simulink model "ES320A_MotDrvDiagc"  (R2013b)
settings: Solver=FixedStepDiscrete  StartTime=0.0  StopTime=1  FixedStep=.002  RelTol=1e-3
undefined symbols (not defined in the file): ARCHGLBPRM_2MILLISEC_SEC_F32, MotDrvDiagcErrFilFrq, MotDrvDiagcErrOffs, MotDrvDiagcErrThd, NtcNr1, NtcSts1, PHAONTISUMMAX_NANOSEC_U32, SysSt1
libraries: simulink x23, Fil x12, NxtrAbslt x6, NxtrLim x6
(part 2 of 3)

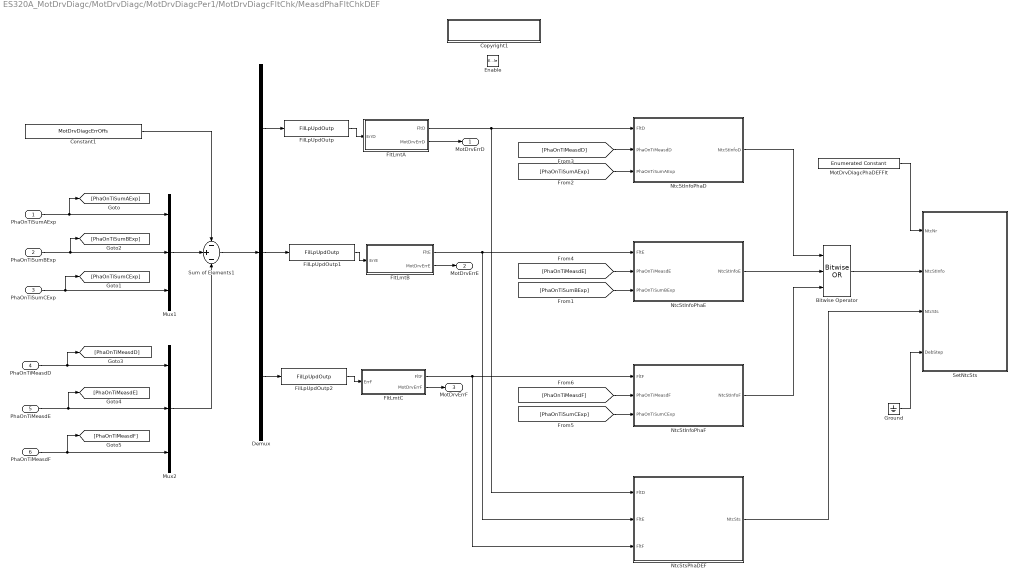
== system ES320A_MotDrvDiagc/MotDrvDiagc/MotDrvDiagcPer1/MotDrvDiagcFltChk/MeasdPhaFltChkDEF ==
  PhaOnTiSumAExp : Inport
  PhaOnTiSumBExp : Inport  Port=2
  PhaOnTiSumCExp : Inport  Port=3
  PhaOnTiMeasdD : Inport  Port=4
  PhaOnTiMeasdE : Inport  Port=5
  PhaOnTiMeasdF : Inport  Port=6
  Enable : EnablePort  StatesWhenEnabling=reset
  Bitwise Operator : simulink/Logic and Bit Operations/Bitwise Operator  logicop=OR  UseBitMask=off  NumInputPorts=3  BitMask=bin2dec('11011001')  BitMaskRealWorld=Stored Integer
  Constant1 : Constant  Value=MotDrvDiagcErrOffs
  Copyright1 : Subsystem  Description=|  RequirementInfo={} %GIDa_58fa1417_7a97_4da9_9225_f2d3186cfd6f  mask(Copyright Information){none=on}
      | Copyright info block.                                               
      |                                                                     
      | Place copyright information at the top of every subsystem in design.
      mask prompts: none "No parameters"
      mask help: Place copyright information at the top of every subsystem in design.
      mask Display:
      | NxtrConf = 'Nexteer Confidential';
      | 
      | sys = bdroot; %handle for the current model ("system")
      | first = get_param(sys,'Created');
      | if(isempty(first))
      |     first = datestr(now,'yyyy');
      | else
      |     first = first(end-3:end);  %year is last four digits
      | end
      | 
      | last = get_param(sys,'LastModifiedDate');
      | if isempty(last)
      |     last = datestr(now,'yyyy');
      | else
      |     last = last(end-3:end);
      | end
      | 
      | if strcmp(first,last)
      |     fprintf('%s\nCopyright  %s Nexteer',NxtrConf,first);
      | else
      |     fprintf('%s\n%s%s-%s Nexteer',NxtrConf,char(169),first,last);
      | end
  Demux : Demux  Outputs=3
  FilLpUpdOutp : Fil/FilLpUpdOutp  StVar=MotDrvDiagcPhaDFilLp
      settings: AttributesFormatString=StVar: %<StVar>
  FilLpUpdOutp1 : Fil/FilLpUpdOutp  StVar=MotDrvDiagcPhaEFilLp
      settings: AttributesFormatString=StVar: %<StVar>
  FilLpUpdOutp2 : Fil/FilLpUpdOutp  StVar=MotDrvDiagcPhaFFilLp
      settings: AttributesFormatString=StVar: %<StVar>
  FltLmtA : Subsystem  RequirementInfo={'linktype_rmi_doors' '0000cf4c (/ESG Group/FDD Module Requirements/EA4 Specific/ES320A_MotDrvDiagc)' '#ES320A_212' 'true' 'REQ: ES320A_212' '' } %GIDa_51d7d654_d101_4f83_80bf_ae722de7e7a9
  FltLmtB : Subsystem  RequirementInfo={'linktype_rmi_doors' '0000cf4c (/ESG Group/FDD Module Requirements/EA4 Specific/ES320A_MotDrvDiagc)' '#ES320A_211' 'true' 'REQ: ES320A_211' '' } %GIDa_eddb3f9b_306c_4d4f_962f_9a75bcde932a
  FltLmtC : Subsystem  RequirementInfo={'linktype_rmi_doors' '0000cf4c (/ESG Group/FDD Module Requirements/EA4 Specific/ES320A_MotDrvDiagc)' '#ES320A_210' 'true' 'REQ: ES320A_210' '' } %GIDa_51c857d3_af1b_4868_8ae8_03f92acada51
  Ground : Ground
  MotDrvDiagcPhaDEFFlt : simulink/Sources/Enumerated Constant  OutDataTypeStr=Enum: NtcNr1  Value=NtcNr1.NTCNR_0X064  SampleTime=inf
  Mux1 : Mux  Inputs=3
  Mux2 : Mux  Inputs=3
  NtcStInfoPhaD : Subsystem
  NtcStInfoPhaE : Subsystem
  NtcStInfoPhaF : Subsystem
  NtcStsPhaDEF : Subsystem  RequirementInfo={'linktype_rmi_doors' '0000cf4c (/ESG Group/FDD Module Requirements/EA4 Specific/ES320A_MotDrvDiagc)' '#ES320A_202' 'true' 'REQ: ES320A_202' '' } %GIDa_66002cee_da6e_4218_8b0a_b4f0ffa61e1a
  SetNtcSts : Subsystem  RequirementInfo={'linktype_rmi_doors' '0000cf4c (/ESG Group/FDD Module Requirements/EA4 Specific/ES320A_MotDrvDiagc)' '#ES320A_159' 'true' 'REQ: ES320A_159' '' } %GIDa_c4017480_1c1a_46e6_ad44_3193a372f033
  Sum of Elements1 : Sum  Inputs=-+-  OutDataTypeStr=single
  MotDrvErrD : Outport
  MotDrvErrE : Outport  Port=2
  MotDrvErrF : Outport  Port=3
  wires:
  FltLmtA/1(FltD) -> NtcStsPhaDEF/1(FltD), NtcStInfoPhaD/1(FltD)
  FltLmtC/1(FltF) -> NtcStsPhaDEF/3(FltF), NtcStInfoPhaF/1(FltF)
  [PhaOnTiMeasdD] -> NtcStInfoPhaD/2(PhaOnTiMeasdD)
  [PhaOnTiSumAExp] -> NtcStInfoPhaD/3(PhaOnTiSumAExp)
  [PhaOnTiMeasdE] -> NtcStInfoPhaE/2(PhaOnTiMeasdE)
  [PhaOnTiSumBExp] -> NtcStInfoPhaE/3(PhaOnTiSumBExp)
  [PhaOnTiMeasdF] -> NtcStInfoPhaF/2(PhaOnTiMeasdF)
  [PhaOnTiSumCExp] -> NtcStInfoPhaF/3(PhaOnTiSumCExp)
  NtcStInfoPhaD/1(NtcStInfoD) -> Bitwise Operator/1
  NtcStInfoPhaE/1(NtcStInfoE) -> Bitwise Operator/2
  NtcStInfoPhaF/1(NtcStInfoF) -> Bitwise Operator/3
  FilLpUpdOutp/1 -> FltLmtA/1(ErrD)
  FilLpUpdOutp2/1 -> FltLmtC/1(ErrF)
  Bitwise Operator/1 -> SetNtcSts/2(NtcStInfo)
  NtcStsPhaDEF/1(NtcSts) -> SetNtcSts/3(NtcSts)
  PhaOnTiMeasdF/1 -> [PhaOnTiMeasdF], Mux2/3
  PhaOnTiMeasdE/1 -> [PhaOnTiMeasdE], Mux2/2
  PhaOnTiMeasdD/1 -> [PhaOnTiMeasdD], Mux2/1
  Constant1/1 -> Sum of Elements1/1
  Mux2/1 -> Sum of Elements1/3
  Sum of Elements1/1 -> Demux/1
  Mux1/1 -> Sum of Elements1/2
  PhaOnTiSumAExp/1 -> [PhaOnTiSumAExp], Mux1/1
  PhaOnTiSumCExp/1 -> [PhaOnTiSumCExp], Mux1/3
  PhaOnTiSumBExp/1 -> [PhaOnTiSumBExp], Mux1/2
  Demux/1 -> FilLpUpdOutp/1
  Demux/2 -> FilLpUpdOutp1/1
  Demux/3 -> FilLpUpdOutp2/1
  Ground/1 -> SetNtcSts/4(DebStep)
  MotDrvDiagcPhaDEFFlt/1 -> SetNtcSts/1(NtcNr)
  FltLmtB/1(FltE) -> NtcStsPhaDEF/2(FltE), NtcStInfoPhaE/1(FltE)
  FilLpUpdOutp1/1 -> FltLmtB/1(ErrE)
  FltLmtA/2(MotDrvErrD) -> MotDrvErrD/1
  FltLmtB/2(MotDrvErrE) -> MotDrvErrE/1
  FltLmtC/2(MotDrvErrF) -> MotDrvErrF/1

== system ES320A_MotDrvDiagc/MotDrvDiagc/MotDrvDiagcPer1/DeltaCompu/else/CopyRight1 ==

== system ES320A_MotDrvDiagc/MotDrvDiagc/MotDrvDiagcPer1/DeltaCompu/else1/CopyRight1 ==

== system ES320A_MotDrvDiagc/MotDrvDiagc/MotDrvDiagcPer1/DeltaCompu/else2/CopyRight1 ==

== system ES320A_MotDrvDiagc/MotDrvDiagc/MotDrvDiagcPer1/DeltaCompu/if/CopyRight1 ==

== system ES320A_MotDrvDiagc/MotDrvDiagc/MotDrvDiagcPer1/DeltaCompu/if1/CopyRight1 ==

== system ES320A_MotDrvDiagc/MotDrvDiagc/MotDrvDiagcPer1/DeltaCompu/if2/CopyRight1 ==

== system ES320A_MotDrvDiagc/MotDrvDiagc/MotDrvDiagcPer1/MotDrvDiagcFltChk/MeasdPhaFltChkABC/Copyright1 ==

== system ES320A_MotDrvDiagc/MotDrvDiagc/MotDrvDiagcPer1/MotDrvDiagcFltChk/MeasdPhaFltChkABC/FltLmtA ==
  ErrA : Inport
  Abslt_f32_f32 : NxtrAbslt/Abslt_f32_f32  SFunctionSpec=single y1 = Abslt_f32_f32(single u1)
      settings: AttributesFormatString=%<Name>
  Constant2 : Constant  Value=MotDrvDiagcErrThd
  Copyright1 : Subsystem  Description=|  RequirementInfo={} %GIDa_ded85060_8e2b_4f15_bbc9_ae7ad683cc8a  mask(Copyright Information){none=on}
      | Copyright info block.                                               
      |                                                                     
      | Place copyright information at the top of every subsystem in design.
      mask prompts: none "No parameters"
      mask help: Place copyright information at the top of every subsystem in design.
      mask Display:
      | NxtrConf = 'Nexteer Confidential';
      | 
      | sys = bdroot; %handle for the current model ("system")
      | first = get_param(sys,'Created');
      | if(isempty(first))
      |     first = datestr(now,'yyyy');
      | else
      |     first = first(end-3:end);  %year is last four digits
      | end
      | 
      | last = get_param(sys,'LastModifiedDate');
      | if isempty(last)
      |     last = datestr(now,'yyyy');
      | else
      |     last = last(end-3:end);
      | end
      | 
      | if strcmp(first,last)
      |     fprintf('%s\nCopyright  %s Nexteer',NxtrConf,first);
      | else
      |     fprintf('%s\n%s%s-%s Nexteer',NxtrConf,char(169),first,last);
      | end
  LimStat_f1 : NxtrLim/LimStat_f32  LoLim=MotDrvErrA.EngMin  HiLim=MotDrvErrA.EngMax
      settings: AttributesFormatString=|
      | Low Limit: %<LoLim>
      | High Limit:%<HiLim>
  Relational Operator : RelationalOperator  Operator=>  OutDataTypeStr=boolean
  FltA : Outport
  MotDrvErrA : Outport  Port=2
  wires:
  ErrA/1 -> Abslt_f32_f32/1
  Constant2/1 -> Relational Operator/2
  Relational Operator/1 -> FltA/1
  Abslt_f32_f32/1 -> LimStat_f1/1, Relational Operator/1
  LimStat_f1/1 -> MotDrvErrA/1

== system ES320A_MotDrvDiagc/MotDrvDiagc/MotDrvDiagcPer1/MotDrvDiagcFltChk/MeasdPhaFltChkABC/FltLmtB ==
  ErrB : Inport
  Abslt_f32_f32 : NxtrAbslt/Abslt_f32_f32  SFunctionSpec=single y1 = Abslt_f32_f32(single u1)
      settings: AttributesFormatString=%<Name>
  Constant2 : Constant  Value=MotDrvDiagcErrThd
  Copyright1 : Subsystem  Description=|  RequirementInfo={} %GIDa_76afdc08_624c_4107_8b02_e46a83163c5b  mask(Copyright Information){none=on}
      | Copyright info block.                                               
      |                                                                     
      | Place copyright information at the top of every subsystem in design.
      mask prompts: none "No parameters"
      mask help: Place copyright information at the top of every subsystem in design.
      mask Display:
      | NxtrConf = 'Nexteer Confidential';
      | 
      | sys = bdroot; %handle for the current model ("system")
      | first = get_param(sys,'Created');
      | if(isempty(first))
      |     first = datestr(now,'yyyy');
      | else
      |     first = first(end-3:end);  %year is last four digits
      | end
      | 
      | last = get_param(sys,'LastModifiedDate');
      | if isempty(last)
      |     last = datestr(now,'yyyy');
      | else
      |     last = last(end-3:end);
      | end
      | 
      | if strcmp(first,last)
      |     fprintf('%s\nCopyright  %s Nexteer',NxtrConf,first);
      | else
      |     fprintf('%s\n%s%s-%s Nexteer',NxtrConf,char(169),first,last);
      | end
  LimStat_f2 : NxtrLim/LimStat_f32  LoLim=MotDrvErrB.EngMin  HiLim=MotDrvErrB.EngMax
      settings: AttributesFormatString=|
      | Low Limit: %<LoLim>
      | High Limit:%<HiLim>
  Relational Operator : RelationalOperator  Operator=>  OutDataTypeStr=boolean
  FltB : Outport
  MotDrvErrB : Outport  Port=2
  wires:
  Relational Operator/1 -> FltB/1
  Constant2/1 -> Relational Operator/2
  Abslt_f32_f32/1 -> LimStat_f2/1, Relational Operator/1
  ErrB/1 -> Abslt_f32_f32/1
  LimStat_f2/1 -> MotDrvErrB/1

== system ES320A_MotDrvDiagc/MotDrvDiagc/MotDrvDiagcPer1/MotDrvDiagcFltChk/MeasdPhaFltChkABC/FltLmtC ==
  ErrC : Inport
  Abslt_f32_f32 : NxtrAbslt/Abslt_f32_f32  SFunctionSpec=single y1 = Abslt_f32_f32(single u1)
      settings: AttributesFormatString=%<Name>
  Constant2 : Constant  Value=MotDrvDiagcErrThd
  Copyright1 : Subsystem  Description=|  RequirementInfo={} %GIDa_37053073_c47e_4fb3_8cd7_4f83c0fb15a4  mask(Copyright Information){none=on}
      | Copyright info block.                                               
      |                                                                     
      | Place copyright information at the top of every subsystem in design.
      mask prompts: none "No parameters"
      mask help: Place copyright information at the top of every subsystem in design.
      mask Display:
      | NxtrConf = 'Nexteer Confidential';
      | 
      | sys = bdroot; %handle for the current model ("system")
      | first = get_param(sys,'Created');
      | if(isempty(first))
      |     first = datestr(now,'yyyy');
      | else
      |     first = first(end-3:end);  %year is last four digits
      | end
      | 
      | last = get_param(sys,'LastModifiedDate');
      | if isempty(last)
      |     last = datestr(now,'yyyy');
      | else
      |     last = last(end-3:end);
      | end
      | 
      | if strcmp(first,last)
      |     fprintf('%s\nCopyright  %s Nexteer',NxtrConf,first);
      | else
      |     fprintf('%s\n%s%s-%s Nexteer',NxtrConf,char(169),first,last);
      | end
  LimStat_f3 : NxtrLim/LimStat_f32  LoLim=MotDrvErrC.EngMin  HiLim=MotDrvErrC.EngMax
      settings: AttributesFormatString=|
      | Low Limit: %<LoLim>
      | High Limit:%<HiLim>
  Relational Operator : RelationalOperator  Operator=>  OutDataTypeStr=boolean
  FltC : Outport
  MotDrvErrC : Outport  Port=2
  wires:
  ErrC/1 -> Abslt_f32_f32/1
  Constant2/1 -> Relational Operator/2
  Relational Operator/1 -> FltC/1
  Abslt_f32_f32/1 -> LimStat_f3/1, Relational Operator/1
  LimStat_f3/1 -> MotDrvErrC/1

== system ES320A_MotDrvDiagc/MotDrvDiagc/MotDrvDiagcPer1/MotDrvDiagcFltChk/MeasdPhaFltChkABC/NtcStInfoPhaA ==
  FltA : Inport
  PhaOnTiMeasdA : Inport  Port=2
  PhaOnTiSumAExp : Inport  Port=3
  Copyright1 : Subsystem  Description=|  RequirementInfo={} %GIDa_f6b7d8fe_5be3_402f_916a_b6caca477132  mask(Copyright Information){none=on}
      | Copyright info block.                                               
      |                                                                     
      | Place copyright information at the top of every subsystem in design.
      mask prompts: none "No parameters"
      mask help: Place copyright information at the top of every subsystem in design.
      mask Display:
      | NxtrConf = 'Nexteer Confidential';
      | 
      | sys = bdroot; %handle for the current model ("system")
      | first = get_param(sys,'Created');
      | if(isempty(first))
      |     first = datestr(now,'yyyy');
      | else
      |     first = first(end-3:end);  %year is last four digits
      | end
      | 
      | last = get_param(sys,'LastModifiedDate');
      | if isempty(last)
      |     last = datestr(now,'yyyy');
      | else
      |     last = last(end-3:end);
      | end
      | 
      | if strcmp(first,last)
      |     fprintf('%s\nCopyright  %s Nexteer',NxtrConf,first);
      | else
      |     fprintf('%s\n%s%s-%s Nexteer',NxtrConf,char(169),first,last);
      | end
  DetermineBitsetA : Subsystem  TreatAsAtomicUnit=on
  DetermineBitsetA1 : Subsystem  RequirementInfo={'linktype_rmi_doors' '0000cf4c (/ESG Group/FDD Module Requirements/EA4 Specific/ES320A_MotDrvDiagc)' '#ES320A_164' 'true' 'REQ: ES320A_164' '' } %GIDa_a157fcae_4dcd_4f05_b388_763736355bda  TreatAsAtomicUnit=on
  If : If  IfExpression=u1 == 1
  Merge : Merge
  NtcStInfoA : Outport
  wires:
  PhaOnTiMeasdA/1 -> DetermineBitsetA/1(PhaOnTiMeasdA)
  DetermineBitsetA1/1(BitSetA) -> Merge/2
  FltA/1 -> If/1
  DetermineBitsetA/1(BitSetA) -> Merge/1
  PhaOnTiSumAExp/1 -> DetermineBitsetA/2(PhaOnTiSumAExp)
  Merge/1 -> NtcStInfoA/1
  If/1 -> DetermineBitsetA/Action
  If/2 -> DetermineBitsetA1/Action

== system ES320A_MotDrvDiagc/MotDrvDiagc/MotDrvDiagcPer1/MotDrvDiagcFltChk/MeasdPhaFltChkABC/NtcStInfoPhaB ==
  FltB : Inport
  PhaOnTiMeasdB : Inport  Port=2
  PhaOnTiSumBExp : Inport  Port=3
  Copyright1 : Subsystem  Description=|  RequirementInfo={} %GIDa_8a865a79_d063_4821_8f7f_5a173239adfd  mask(Copyright Information){none=on}
      | Copyright info block.                                               
      |                                                                     
      | Place copyright information at the top of every subsystem in design.
      mask prompts: none "No parameters"
      mask help: Place copyright information at the top of every subsystem in design.
      mask Display:
      | NxtrConf = 'Nexteer Confidential';
      | 
      | sys = bdroot; %handle for the current model ("system")
      | first = get_param(sys,'Created');
      | if(isempty(first))
      |     first = datestr(now,'yyyy');
      | else
      |     first = first(end-3:end);  %year is last four digits
      | end
      | 
      | last = get_param(sys,'LastModifiedDate');
      | if isempty(last)
      |     last = datestr(now,'yyyy');
      | else
      |     last = last(end-3:end);
      | end
      | 
      | if strcmp(first,last)
      |     fprintf('%s\nCopyright  %s Nexteer',NxtrConf,first);
      | else
      |     fprintf('%s\n%s%s-%s Nexteer',NxtrConf,char(169),first,last);
      | end
  DetermineBitsetB : Subsystem  TreatAsAtomicUnit=on
  DetermineBitsetB1 : Subsystem  RequirementInfo={'linktype_rmi_doors' '0000cf4c (/ESG Group/FDD Module Requirements/EA4 Specific/ES320A_MotDrvDiagc)' '#ES320A_164' 'true' 'REQ: ES320A_164' '' } %GIDa_ef53c142_7f27_4df6_aa45_b15ec14132a0  TreatAsAtomicUnit=on
  If : If  IfExpression=u1 == 1
  Merge : Merge
  NtcStInfoB : Outport
  wires:
  DetermineBitsetB1/1(BitSetB) -> Merge/2
  FltB/1 -> If/1
  PhaOnTiSumBExp/1 -> DetermineBitsetB/2(PhaOnTiSumBExp)
  PhaOnTiMeasdB/1 -> DetermineBitsetB/1(PhaOnTiMeasdB)
  Merge/1 -> NtcStInfoB/1
  DetermineBitsetB/1(BitSetB) -> Merge/1
  If/1 -> DetermineBitsetB/Action
  If/2 -> DetermineBitsetB1/Action

== system ES320A_MotDrvDiagc/MotDrvDiagc/MotDrvDiagcPer1/MotDrvDiagcFltChk/MeasdPhaFltChkABC/NtcStInfoPhaC ==
  FltC : Inport
  PhaOnTiMeasdC : Inport  Port=2
  PhaOnTiSumCExp : Inport  Port=3
  Copyright1 : Subsystem  Description=|  RequirementInfo={} %GIDa_1949ea6a_a67d_400f_aabf_09f17ca06aa3  mask(Copyright Information){none=on}
      | Copyright info block.                                               
      |                                                                     
      | Place copyright information at the top of every subsystem in design.
      mask prompts: none "No parameters"
      mask help: Place copyright information at the top of every subsystem in design.
      mask Display:
      | NxtrConf = 'Nexteer Confidential';
      | 
      | sys = bdroot; %handle for the current model ("system")
      | first = get_param(sys,'Created');
      | if(isempty(first))
      |     first = datestr(now,'yyyy');
      | else
      |     first = first(end-3:end);  %year is last four digits
      | end
      | 
      | last = get_param(sys,'LastModifiedDate');
      | if isempty(last)
      |     last = datestr(now,'yyyy');
      | else
      |     last = last(end-3:end);
      | end
      | 
      | if strcmp(first,last)
      |     fprintf('%s\nCopyright  %s Nexteer',NxtrConf,first);
      | else
      |     fprintf('%s\n%s%s-%s Nexteer',NxtrConf,char(169),first,last);
      | end
  DetermineBitsetC : Subsystem  TreatAsAtomicUnit=on
  DetermineBitsetC1 : Subsystem  RequirementInfo={'linktype_rmi_doors' '0000cf4c (/ESG Group/FDD Module Requirements/EA4 Specific/ES320A_MotDrvDiagc)' '#ES320A_164' 'true' 'REQ: ES320A_164' '' } %GIDa_512545ae_b061_4cfd_bb08_eb9229f95692  TreatAsAtomicUnit=on
  If : If  IfExpression=u1 == 1
  Merge : Merge
  NtcStInfoC : Outport
  wires:
  FltC/1 -> If/1
  PhaOnTiSumCExp/1 -> DetermineBitsetC/2(PhaOnTiSumCExp)
  PhaOnTiMeasdC/1 -> DetermineBitsetC/1(PhaOnTiMeasdC)
  DetermineBitsetC/1(BitSetC) -> Merge/1
  DetermineBitsetC1/1(BitSetC) -> Merge/2
  Merge/1 -> NtcStInfoC/1
  If/1 -> DetermineBitsetC/Action
  If/2 -> DetermineBitsetC1/Action

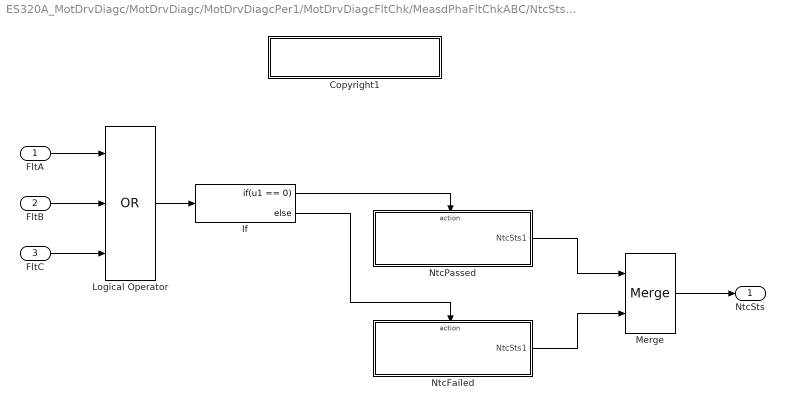
== system ES320A_MotDrvDiagc/MotDrvDiagc/MotDrvDiagcPer1/MotDrvDiagcFltChk/MeasdPhaFltChkABC/NtcStsPhaABC ==
  FltA : Inport
  FltB : Inport  Port=2
  FltC : Inport  Port=3
  Copyright1 : Subsystem  Description=|  RequirementInfo={} %GIDa_bbf24996_5a5d_487b_b234_27f9deb21f2d  mask(Copyright Information){none=on}
      | Copyright info block.                                               
      |                                                                     
      | Place copyright information at the top of every subsystem in design.
      mask prompts: none "No parameters"
      mask help: Place copyright information at the top of every subsystem in design.
      mask Display:
      | NxtrConf = 'Nexteer Confidential';
      | 
      | sys = bdroot; %handle for the current model ("system")
      | first = get_param(sys,'Created');
      | if(isempty(first))
      |     first = datestr(now,'yyyy');
      | else
      |     first = first(end-3:end);  %year is last four digits
      | end
      | 
      | last = get_param(sys,'LastModifiedDate');
      | if isempty(last)
      |     last = datestr(now,'yyyy');
      | else
      |     last = last(end-3:end);
      | end
      | 
      | if strcmp(first,last)
      |     fprintf('%s\nCopyright  %s Nexteer',NxtrConf,first);
      | else
      |     fprintf('%s\n%s%s-%s Nexteer',NxtrConf,char(169),first,last);
      | end
  If : If  IfExpression=u1 == 0
  Logical Operator : Logic  Operator=OR  Inputs=3  AllPortsSameDT=off  OutDataTypeStr=boolean
  Merge : Merge
  NtcFailed : Subsystem  TreatAsAtomicUnit=on
  NtcPassed : Subsystem  TreatAsAtomicUnit=on
  NtcSts : Outport
  wires:
  NtcFailed/1(NtcSts1) -> Merge/2
  Merge/1 -> NtcSts/1
  FltC/1 -> Logical Operator/3
  If/2 -> NtcFailed/Action
  FltB/1 -> Logical Operator/2
  FltA/1 -> Logical Operator/1
  NtcPassed/1(NtcSts1) -> Merge/1
  Logical Operator/1 -> If/1
  If/1 -> NtcPassed/Action

== system ES320A_MotDrvDiagc/MotDrvDiagc/MotDrvDiagcPer1/MotDrvDiagcFltChk/MeasdPhaFltChkABC/SetNtcSts ==
  NtcNr : Inport
  NtcStInfo : Inport  Port=2
  NtcSts : Inport  Port=3
  DebStep : Inport  Port=4
  Copyright1 : Subsystem  Description=|  RequirementInfo={} %GIDa_12d57861_183b_4f8f_9d75_9f3f69d3d00b  mask(Copyright Information){none=on}
      | Copyright info block.                                               
      |                                                                     
      | Place copyright information at the top of every subsystem in design.
      mask prompts: none "No parameters"
      mask help: Place copyright information at the top of every subsystem in design.
      mask Display:
      | NxtrConf = 'Nexteer Confidential';
      | 
      | sys = bdroot; %handle for the current model ("system")
      | first = get_param(sys,'Created');
      | if(isempty(first))
      |     first = datestr(now,'yyyy');
      | else
      |     first = first(end-3:end);  %year is last four digits
      | end
      | 
      | last = get_param(sys,'LastModifiedDate');
      | if isempty(last)
      |     last = datestr(now,'yyyy');
      | else
      |     last = last(end-3:end);
      | end
      | 
      | if strcmp(first,last)
      |     fprintf('%s\nCopyright  %s Nexteer',NxtrConf,first);
      | else
      |     fprintf('%s\n%s%s-%s Nexteer',NxtrConf,char(169),first,last);
      | end
  Data Store Write : DataStoreWrite  DataStoreName=Ntc0x054StsVal
  Data Store Write1 : DataStoreWrite  DataStoreName=Ntc0x054StsInfoVal
  Data Store Write2 : DataStoreWrite  DataStoreName=Ntc0x054Nr
  Terminator2 : Terminator
  wires:
  NtcNr/1 -> Data Store Write2/1
  NtcStInfo/1 -> Data Store Write1/1
  DebStep/1 -> Terminator2/1
  NtcSts/1 -> Data Store Write/1

== system ES320A_MotDrvDiagc/MotDrvDiagc/MotDrvDiagcPer1/MotDrvDiagcFltChk/MeasdPhaFltChkDEF/Copyright1 ==

== system ES320A_MotDrvDiagc/MotDrvDiagc/MotDrvDiagcPer1/MotDrvDiagcFltChk/MeasdPhaFltChkDEF/FltLmtA ==
  ErrD : Inport
  Abslt_f32_f32 : NxtrAbslt/Abslt_f32_f32  SFunctionSpec=single y1 = Abslt_f32_f32(single u1)
      settings: AttributesFormatString=%<Name>
  Constant2 : Constant  Value=MotDrvDiagcErrThd
  Copyright1 : Subsystem  Description=|  RequirementInfo={} %GIDa_c8d3461b_e8b8_48e5_b0de_d035927cdfa4  mask(Copyright Information){none=on}
      | Copyright info block.                                               
      |                                                                     
      | Place copyright information at the top of every subsystem in design.
      mask prompts: none "No parameters"
      mask help: Place copyright information at the top of every subsystem in design.
      mask Display:
      | NxtrConf = 'Nexteer Confidential';
      | 
      | sys = bdroot; %handle for the current model ("system")
      | first = get_param(sys,'Created');
      | if(isempty(first))
      |     first = datestr(now,'yyyy');
      | else
      |     first = first(end-3:end);  %year is last four digits
      | end
      | 
      | last = get_param(sys,'LastModifiedDate');
      | if isempty(last)
      |     last = datestr(now,'yyyy');
      | else
      |     last = last(end-3:end);
      | end
      | 
      | if strcmp(first,last)
      |     fprintf('%s\nCopyright  %s Nexteer',NxtrConf,first);
      | else
      |     fprintf('%s\n%s%s-%s Nexteer',NxtrConf,char(169),first,last);
      | end
  LimStat_f3 : NxtrLim/LimStat_f32  LoLim=MotDrvErrD.EngMin  HiLim=MotDrvErrD.EngMax
      settings: AttributesFormatString=|
      | Low Limit: %<LoLim>
      | High Limit:%<HiLim>
  Relational Operator : RelationalOperator  Operator=>  OutDataTypeStr=boolean
  FltD : Outport
  MotDrvErrD : Outport  Port=2
  wires:
  ErrD/1 -> Abslt_f32_f32/1
  Constant2/1 -> Relational Operator/2
  Relational Operator/1 -> FltD/1
  Abslt_f32_f32/1 -> LimStat_f3/1, Relational Operator/1
  LimStat_f3/1 -> MotDrvErrD/1

== system ES320A_MotDrvDiagc/MotDrvDiagc/MotDrvDiagcPer1/MotDrvDiagcFltChk/MeasdPhaFltChkDEF/FltLmtB ==
  ErrE : Inport
  Abslt_f32_f32 : NxtrAbslt/Abslt_f32_f32  SFunctionSpec=single y1 = Abslt_f32_f32(single u1)
      settings: AttributesFormatString=%<Name>
  Constant2 : Constant  Value=MotDrvDiagcErrThd
  Copyright1 : Subsystem  Description=|  RequirementInfo={} %GIDa_af57eb4c_60cb_4d89_abbc_1a0b8ab95bfa  mask(Copyright Information){none=on}
      | Copyright info block.                                               
      |                                                                     
      | Place copyright information at the top of every subsystem in design.
      mask prompts: none "No parameters"
      mask help: Place copyright information at the top of every subsystem in design.
      mask Display:
      | NxtrConf = 'Nexteer Confidential';
      | 
      | sys = bdroot; %handle for the current model ("system")
      | first = get_param(sys,'Created');
      | if(isempty(first))
      |     first = datestr(now,'yyyy');
      | else
      |     first = first(end-3:end);  %year is last four digits
      | end
      | 
      | last = get_param(sys,'LastModifiedDate');
      | if isempty(last)
      |     last = datestr(now,'yyyy');
      | else
      |     last = last(end-3:end);
      | end
      | 
      | if strcmp(first,last)
      |     fprintf('%s\nCopyright  %s Nexteer',NxtrConf,first);
      | else
      |     fprintf('%s\n%s%s-%s Nexteer',NxtrConf,char(169),first,last);
      | end
  LimStat_f1 : NxtrLim/LimStat_f32  LoLim=MotDrvErrE.EngMin  HiLim=MotDrvErrE.EngMax
      settings: AttributesFormatString=|
      | Low Limit: %<LoLim>
      | High Limit:%<HiLim>
  Relational Operator : RelationalOperator  Operator=>  OutDataTypeStr=boolean
  FltE : Outport
  MotDrvErrE : Outport  Port=2
  wires:
  Relational Operator/1 -> FltE/1
  Constant2/1 -> Relational Operator/2
  Abslt_f32_f32/1 -> LimStat_f1/1, Relational Operator/1
  ErrE/1 -> Abslt_f32_f32/1
  LimStat_f1/1 -> MotDrvErrE/1

== system ES320A_MotDrvDiagc/MotDrvDiagc/MotDrvDiagcPer1/MotDrvDiagcFltChk/MeasdPhaFltChkDEF/FltLmtC ==
  ErrF : Inport
  Abslt_f32_f32 : NxtrAbslt/Abslt_f32_f32  SFunctionSpec=single y1 = Abslt_f32_f32(single u1)
      settings: AttributesFormatString=%<Name>
  Constant2 : Constant  Value=MotDrvDiagcErrThd
  Copyright1 : Subsystem  Description=|  RequirementInfo={} %GIDa_c95a8031_7a3f_460e_8aef_15bdbfe2c2c0  mask(Copyright Information){none=on}
      | Copyright info block.                                               
      |                                                                     
      | Place copyright information at the top of every subsystem in design.
      mask prompts: none "No parameters"
      mask help: Place copyright information at the top of every subsystem in design.
      mask Display:
      | NxtrConf = 'Nexteer Confidential';
      | 
      | sys = bdroot; %handle for the current model ("system")
      | first = get_param(sys,'Created');
      | if(isempty(first))
      |     first = datestr(now,'yyyy');
      | else
      |     first = first(end-3:end);  %year is last four digits
      | end
      | 
      | last = get_param(sys,'LastModifiedDate');
      | if isempty(last)
      |     last = datestr(now,'yyyy');
      | else
      |     last = last(end-3:end);
      | end
      | 
      | if strcmp(first,last)
      |     fprintf('%s\nCopyright  %s Nexteer',NxtrConf,first);
      | else
      |     fprintf('%s\n%s%s-%s Nexteer',NxtrConf,char(169),first,last);
      | end
  LimStat_f2 : NxtrLim/LimStat_f32  LoLim=MotDrvErrF.EngMin  HiLim=MotDrvErrF.EngMax
      settings: AttributesFormatString=|
      | Low Limit: %<LoLim>
      | High Limit:%<HiLim>
  Relational Operator : RelationalOperator  Operator=>  OutDataTypeStr=boolean
  FltF : Outport
  MotDrvErrF : Outport  Port=2
  wires:
  ErrF/1 -> Abslt_f32_f32/1
  Abslt_f32_f32/1 -> LimStat_f2/1, Relational Operator/1
  Constant2/1 -> Relational Operator/2
  Relational Operator/1 -> FltF/1
  LimStat_f2/1 -> MotDrvErrF/1

== system ES320A_MotDrvDiagc/MotDrvDiagc/MotDrvDiagcPer1/MotDrvDiagcFltChk/MeasdPhaFltChkDEF/NtcStInfoPhaD ==
  FltD : Inport
  PhaOnTiMeasdD : Inport  Port=2
  PhaOnTiSumAExp : Inport  Port=3
  Copyright1 : Subsystem  Description=|  RequirementInfo={} %GIDa_9dd4480d_c3d9_4f50_b0ad_c73d2515bc03  mask(Copyright Information){none=on}
      | Copyright info block.                                               
      |                                                                     
      | Place copyright information at the top of every subsystem in design.
      mask prompts: none "No parameters"
      mask help: Place copyright information at the top of every subsystem in design.
      mask Display:
      | NxtrConf = 'Nexteer Confidential';
      | 
      | sys = bdroot; %handle for the current model ("system")
      | first = get_param(sys,'Created');
      | if(isempty(first))
      |     first = datestr(now,'yyyy');
      | else
      |     first = first(end-3:end);  %year is last four digits
      | end
      | 
      | last = get_param(sys,'LastModifiedDate');
      | if isempty(last)
      |     last = datestr(now,'yyyy');
      | else
      |     last = last(end-3:end);
      | end
      | 
      | if strcmp(first,last)
      |     fprintf('%s\nCopyright  %s Nexteer',NxtrConf,first);
      | else
      |     fprintf('%s\n%s%s-%s Nexteer',NxtrConf,char(169),first,last);
      | end
  DetermineBitsetD : Subsystem  TreatAsAtomicUnit=on
  DetermineBitsetD1 : Subsystem  RequirementInfo={'linktype_rmi_doors' '0000cf4c (/ESG Group/FDD Module Requirements/EA4 Specific/ES320A_MotDrvDiagc)' '#ES320A_166' 'true' 'REQ: ES320A_166' '' } %GIDa_4f537968_8662_4f52_acc4_881aed44273d  TreatAsAtomicUnit=on
  If : If  IfExpression=u1 == 1
  Merge : Merge
  NtcStInfoD : Outport
  wires:
  PhaOnTiMeasdD/1 -> DetermineBitsetD/1(PhaOnTiMeasdD)
  DetermineBitsetD1/1(BitSetD) -> Merge/2
  FltD/1 -> If/1
  DetermineBitsetD/1(BitSetD) -> Merge/1
  PhaOnTiSumAExp/1 -> DetermineBitsetD/2(PhaOnTiSumAExp)
  Merge/1 -> NtcStInfoD/1
  If/1 -> DetermineBitsetD/Action
  If/2 -> DetermineBitsetD1/Action

== system ES320A_MotDrvDiagc/MotDrvDiagc/MotDrvDiagcPer1/MotDrvDiagcFltChk/MeasdPhaFltChkDEF/NtcStInfoPhaE ==
  FltE : Inport
  PhaOnTiMeasdE : Inport  Port=2
  PhaOnTiSumBExp : Inport  Port=3
  Copyright1 : Subsystem  Description=|  RequirementInfo={} %GIDa_e39717d9_939f_4854_a46a_c13e9cb1fcb5  mask(Copyright Information){none=on}
      | Copyright info block.                                               
      |                                                                     
      | Place copyright information at the top of every subsystem in design.
      mask prompts: none "No parameters"
      mask help: Place copyright information at the top of every subsystem in design.
      mask Display:
      | NxtrConf = 'Nexteer Confidential';
      | 
      | sys = bdroot; %handle for the current model ("system")
      | first = get_param(sys,'Created');
      | if(isempty(first))
      |     first = datestr(now,'yyyy');
      | else
      |     first = first(end-3:end);  %year is last four digits
      | end
      | 
      | last = get_param(sys,'LastModifiedDate');
      | if isempty(last)
      |     last = datestr(now,'yyyy');
      | else
      |     last = last(end-3:end);
      | end
      | 
      | if strcmp(first,last)
      |     fprintf('%s\nCopyright  %s Nexteer',NxtrConf,first);
      | else
      |     fprintf('%s\n%s%s-%s Nexteer',NxtrConf,char(169),first,last);
      | end
  DetermineBitsetE : Subsystem  TreatAsAtomicUnit=on
  DetermineBitsetE1 : Subsystem  RequirementInfo={'linktype_rmi_doors' '0000cf4c (/ESG Group/FDD Module Requirements/EA4 Specific/ES320A_MotDrvDiagc)' '#ES320A_166' 'true' 'REQ: ES320A_166' '' } %GIDa_758e8cb3_9839_4351_bc8b_1d599a210db9  TreatAsAtomicUnit=on
  If : If  IfExpression=u1 == 1
  Merge : Merge
  NtcStInfoE : Outport
  wires:
  DetermineBitsetE1/1(BitSetE) -> Merge/2
  FltE/1 -> If/1
  PhaOnTiSumBExp/1 -> DetermineBitsetE/2(PhaOnTiSumBExp)
  PhaOnTiMeasdE/1 -> DetermineBitsetE/1(PhaOnTiMeasdE)
  Merge/1 -> NtcStInfoE/1
  DetermineBitsetE/1(BitSetE) -> Merge/1
  If/1 -> DetermineBitsetE/Action
  If/2 -> DetermineBitsetE1/Action

== system ES320A_MotDrvDiagc/MotDrvDiagc/MotDrvDiagcPer1/MotDrvDiagcFltChk/MeasdPhaFltChkDEF/NtcStInfoPhaF ==
  FltF : Inport
  PhaOnTiMeasdF : Inport  Port=2
  PhaOnTiSumCExp : Inport  Port=3
  Copyright1 : Subsystem  Description=|  RequirementInfo={} %GIDa_bcf80c75_4c32_4378_a699_a2f19adb34e9  mask(Copyright Information){none=on}
      | Copyright info block.                                               
      |                                                                     
      | Place copyright information at the top of every subsystem in design.
      mask prompts: none "No parameters"
      mask help: Place copyright information at the top of every subsystem in design.
      mask Display:
      | NxtrConf = 'Nexteer Confidential';
      | 
      | sys = bdroot; %handle for the current model ("system")
      | first = get_param(sys,'Created');
      | if(isempty(first))
      |     first = datestr(now,'yyyy');
      | else
      |     first = first(end-3:end);  %year is last four digits
      | end
      | 
      | last = get_param(sys,'LastModifiedDate');
      | if isempty(last)
      |     last = datestr(now,'yyyy');
      | else
      |     last = last(end-3:end);
      | end
      | 
      | if strcmp(first,last)
      |     fprintf('%s\nCopyright  %s Nexteer',NxtrConf,first);
      | else
      |     fprintf('%s\n%s%s-%s Nexteer',NxtrConf,char(169),first,last);
      | end
  DetermineBitsetF : Subsystem  TreatAsAtomicUnit=on
  DetermineBitsetF1 : Subsystem  RequirementInfo={'linktype_rmi_doors' '0000cf4c (/ESG Group/FDD Module Requirements/EA4 Specific/ES320A_MotDrvDiagc)' '#ES320A_166' 'true' 'REQ: ES320A_166' '' } %GIDa_f76cb311_6733_4d7e_8cbe_4f09f5ba5362  TreatAsAtomicUnit=on
  If : If  IfExpression=u1 == 1
  Merge : Merge
  NtcStInfoF : Outport
  wires:
  FltF/1 -> If/1
  PhaOnTiSumCExp/1 -> DetermineBitsetF/2(PhaOnTiSumCExp)
  PhaOnTiMeasdF/1 -> DetermineBitsetF/1(PhaOnTiMeasdF)
  DetermineBitsetF/1(BitSetF) -> Merge/1
  DetermineBitsetF1/1(BitSetF) -> Merge/2
  Merge/1 -> NtcStInfoF/1
  If/1 -> DetermineBitsetF/Action
  If/2 -> DetermineBitsetF1/Action

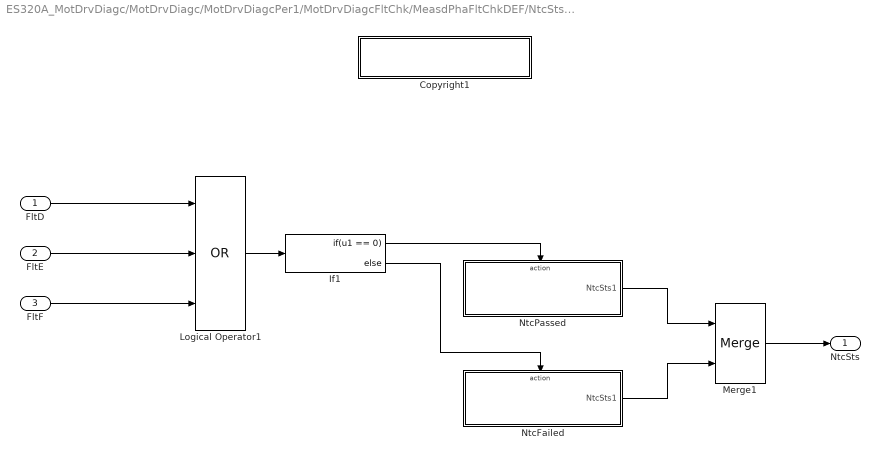
== system ES320A_MotDrvDiagc/MotDrvDiagc/MotDrvDiagcPer1/MotDrvDiagcFltChk/MeasdPhaFltChkDEF/NtcStsPhaDEF ==
  FltD : Inport
  FltE : Inport  Port=2
  FltF : Inport  Port=3
  Copyright1 : Subsystem  Description=|  RequirementInfo={} %GIDa_3e001955_6d0c_4ba7_8891_07e5c461d61f  mask(Copyright Information){none=on}
      | Copyright info block.                                               
      |                                                                     
      | Place copyright information at the top of every subsystem in design.
      mask prompts: none "No parameters"
      mask help: Place copyright information at the top of every subsystem in design.
      mask Display:
      | NxtrConf = 'Nexteer Confidential';
      | 
      | sys = bdroot; %handle for the current model ("system")
      | first = get_param(sys,'Created');
      | if(isempty(first))
      |     first = datestr(now,'yyyy');
      | else
      |     first = first(end-3:end);  %year is last four digits
      | end
      | 
      | last = get_param(sys,'LastModifiedDate');
      | if isempty(last)
      |     last = datestr(now,'yyyy');
      | else
      |     last = last(end-3:end);
      | end
      | 
      | if strcmp(first,last)
      |     fprintf('%s\nCopyright  %s Nexteer',NxtrConf,first);
      | else
      |     fprintf('%s\n%s%s-%s Nexteer',NxtrConf,char(169),first,last);
      | end
  If1 : If  IfExpression=u1 == 0
  Logical Operator1 : Logic  Operator=OR  Inputs=3  AllPortsSameDT=off  OutDataTypeStr=boolean
  Merge1 : Merge
  NtcFailed : Subsystem  TreatAsAtomicUnit=on
  NtcPassed : Subsystem  TreatAsAtomicUnit=on
  NtcSts : Outport
  wires:
  FltF/1 -> Logical Operator1/3
  FltE/1 -> Logical Operator1/2
  FltD/1 -> Logical Operator1/1
  NtcFailed/1(NtcSts1) -> Merge1/2
  Merge1/1 -> NtcSts/1
  If1/2 -> NtcFailed/Action
  NtcPassed/1(NtcSts1) -> Merge1/1
  Logical Operator1/1 -> If1/1
  If1/1 -> NtcPassed/Action

== system ES320A_MotDrvDiagc/MotDrvDiagc/MotDrvDiagcPer1/MotDrvDiagcFltChk/MeasdPhaFltChkDEF/SetNtcSts ==
  NtcNr : Inport
  NtcStInfo : Inport  Port=2
  NtcSts : Inport  Port=3
  DebStep : Inport  Port=4
  Copyright1 : Subsystem  Description=|  RequirementInfo={} %GIDa_82ab73fc_70d3_4000_94b6_c539a339ca25  mask(Copyright Information){none=on}
      | Copyright info block.                                               
      |                                                                     
      | Place copyright information at the top of every subsystem in design.
      mask prompts: none "No parameters"
      mask help: Place copyright information at the top of every subsystem in design.
      mask Display:
      | NxtrConf = 'Nexteer Confidential';
      | 
      | sys = bdroot; %handle for the current model ("system")
      | first = get_param(sys,'Created');
      | if(isempty(first))
      |     first = datestr(now,'yyyy');
      | else
      |     first = first(end-3:end);  %year is last four digits
      | end
      | 
      | last = get_param(sys,'LastModifiedDate');
      | if isempty(last)
      |     last = datestr(now,'yyyy');
      | else
      |     last = last(end-3:end);
      | end
      | 
      | if strcmp(first,last)
      |     fprintf('%s\nCopyright  %s Nexteer',NxtrConf,first);
      | else
      |     fprintf('%s\n%s%s-%s Nexteer',NxtrConf,char(169),first,last);
      | end
  Data Store Write : DataStoreWrite  DataStoreName=Ntc0x064StsVal
  Data Store Write1 : DataStoreWrite  DataStoreName=Ntc0x064StsInfoVal
  Data Store Write2 : DataStoreWrite  DataStoreName=Ntc0x064Nr
  Terminator3 : Terminator
  wires:
  NtcNr/1 -> Data Store Write2/1
  NtcStInfo/1 -> Data Store Write1/1
  NtcSts/1 -> Data Store Write/1
  DebStep/1 -> Terminator3/1

== system ES320A_MotDrvDiagc/MotDrvDiagc/MotDrvDiagcPer1/MotDrvDiagcFltChk/MeasdPhaFltChkABC/FltLmtA/Copyright1 ==

== system ES320A_MotDrvDiagc/MotDrvDiagc/MotDrvDiagcPer1/MotDrvDiagcFltChk/MeasdPhaFltChkABC/FltLmtB/Copyright1 ==

== system ES320A_MotDrvDiagc/MotDrvDiagc/MotDrvDiagcPer1/MotDrvDiagcFltChk/MeasdPhaFltChkABC/FltLmtC/Copyright1 ==

== system ES320A_MotDrvDiagc/MotDrvDiagc/MotDrvDiagcPer1/MotDrvDiagcFltChk/MeasdPhaFltChkABC/NtcStInfoPhaA/Copyright1 ==

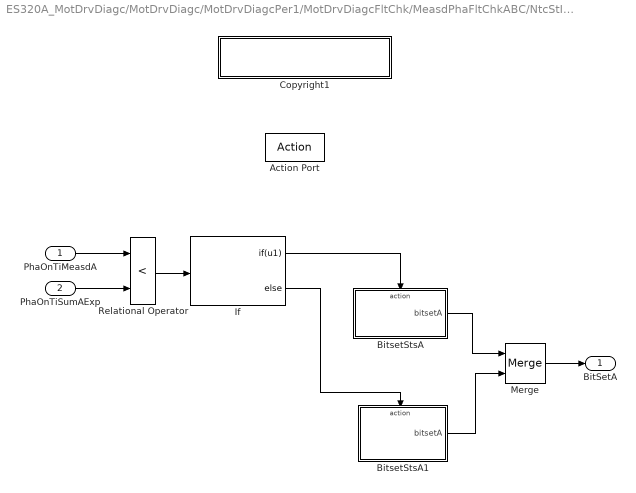
== system ES320A_MotDrvDiagc/MotDrvDiagc/MotDrvDiagcPer1/MotDrvDiagcFltChk/MeasdPhaFltChkABC/NtcStInfoPhaA/DetermineBitsetA ==
  PhaOnTiMeasdA : Inport
  PhaOnTiSumAExp : Inport  Port=2
  Action Port : ActionPort  ActionType=then
  BitsetStsA : Subsystem  RequirementInfo={'linktype_rmi_doors' '0000cf4c (/ESG Group/FDD Module Requirements/EA4 Specific/ES320A_MotDrvDiagc)' '#ES320A_163' 'true' 'REQ: ES320A_163' '' } %GIDa_67335626_7f3e_46bc_927b_f434e3db3a69  TreatAsAtomicUnit=on
  BitsetStsA1 : Subsystem  RequirementInfo={'linktype_rmi_doors' '0000cf4c (/ESG Group/FDD Module Requirements/EA4 Specific/ES320A_MotDrvDiagc)' '#ES320A_194' 'true' 'REQ: ES320A_194' '' } %GIDa_39899d30_c943_4541_a011_39acdbdd3e79  TreatAsAtomicUnit=on
  Copyright1 : Subsystem  Description=|  RequirementInfo={} %GIDa_b2068767_f8c2_42e3_88ee_b71c1895a0fe  mask(Copyright Information){none=on}
      | Copyright info block.                                               
      |                                                                     
      | Place copyright information at the top of every subsystem in design.
      mask prompts: none "No parameters"
      mask help: Place copyright information at the top of every subsystem in design.
      mask Display:
      | NxtrConf = 'Nexteer Confidential';
      | 
      | sys = bdroot; %handle for the current model ("system")
      | first = get_param(sys,'Created');
      | if(isempty(first))
      |     first = datestr(now,'yyyy');
      | else
      |     first = first(end-3:end);  %year is last four digits
      | end
      | 
      | last = get_param(sys,'LastModifiedDate');
      | if isempty(last)
      |     last = datestr(now,'yyyy');
      | else
      |     last = last(end-3:end);
      | end
      | 
      | if strcmp(first,last)
      |     fprintf('%s\nCopyright  %s Nexteer',NxtrConf,first);
      | else
      |     fprintf('%s\n%s%s-%s Nexteer',NxtrConf,char(169),first,last);
      | end
  If : If  IfExpression=u1
  Merge : Merge
  Relational Operator : RelationalOperator  Operator=<  OutDataTypeStr=boolean
  BitSetA : Outport
  wires:
  BitsetStsA/1(bitsetA) -> Merge/1
  BitsetStsA1/1(bitsetA) -> Merge/2
  Merge/1 -> BitSetA/1
  If/1 -> BitsetStsA/Action
  If/2 -> BitsetStsA1/Action
  Relational Operator/1 -> If/1
  PhaOnTiMeasdA/1 -> Relational Operator/1
  PhaOnTiSumAExp/1 -> Relational Operator/2

== system ES320A_MotDrvDiagc/MotDrvDiagc/MotDrvDiagcPer1/MotDrvDiagcFltChk/MeasdPhaFltChkABC/NtcStInfoPhaA/DetermineBitsetA1 ==
  Action Port : ActionPort  ActionType=else
  Constant5 : Constant  Value=0  OutDataTypeStr=uint8
  Copyright1 : Subsystem  Description=|  RequirementInfo={} %GIDa_7eab0cbe_b26a_4140_b851_773438c6c4cc  mask(Copyright Information){none=on}
      | Copyright info block.                                               
      |                                                                     
      | Place copyright information at the top of every subsystem in design.
      mask prompts: none "No parameters"
      mask help: Place copyright information at the top of every subsystem in design.
      mask Display:
      | NxtrConf = 'Nexteer Confidential';
      | 
      | sys = bdroot; %handle for the current model ("system")
      | first = get_param(sys,'Created');
      | if(isempty(first))
      |     first = datestr(now,'yyyy');
      | else
      |     first = first(end-3:end);  %year is last four digits
      | end
      | 
      | last = get_param(sys,'LastModifiedDate');
      | if isempty(last)
      |     last = datestr(now,'yyyy');
      | else
      |     last = last(end-3:end);
      | end
      | 
      | if strcmp(first,last)
      |     fprintf('%s\nCopyright  %s Nexteer',NxtrConf,first);
      | else
      |     fprintf('%s\n%s%s-%s Nexteer',NxtrConf,char(169),first,last);
      | end
  BitSetA : Outport
  wires:
  Constant5/1 -> BitSetA/1

== system ES320A_MotDrvDiagc/MotDrvDiagc/MotDrvDiagcPer1/MotDrvDiagcFltChk/MeasdPhaFltChkABC/NtcStInfoPhaB/Copyright1 ==

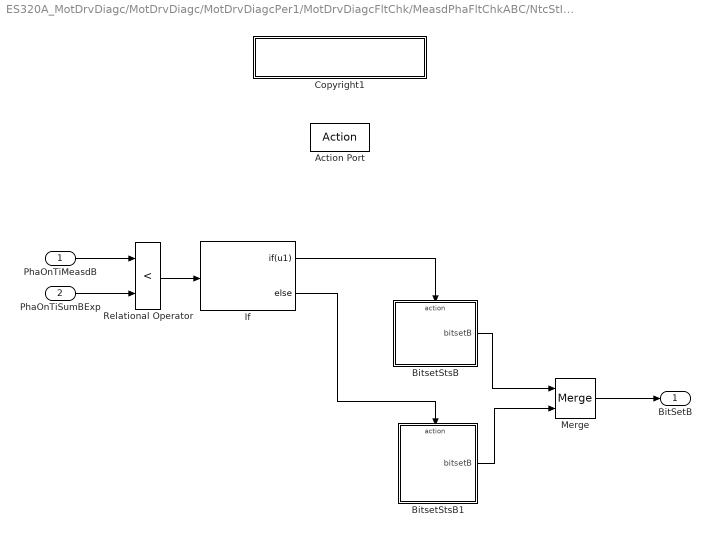
== system ES320A_MotDrvDiagc/MotDrvDiagc/MotDrvDiagcPer1/MotDrvDiagcFltChk/MeasdPhaFltChkABC/NtcStInfoPhaB/DetermineBitsetB ==
  PhaOnTiMeasdB : Inport
  PhaOnTiSumBExp : Inport  Port=2
  Action Port : ActionPort  ActionType=then
  BitsetStsB : Subsystem  RequirementInfo={'linktype_rmi_doors' '0000cf4c (/ESG Group/FDD Module Requirements/EA4 Specific/ES320A_MotDrvDiagc)' '#ES320A_193' 'true' 'REQ: ES320A_193' '' } %GIDa_de542b76_80c4_4bcb_ac8c_b0c66a31fa88  TreatAsAtomicUnit=on
  BitsetStsB1 : Subsystem  RequirementInfo={'linktype_rmi_doors' '0000cf4c (/ESG Group/FDD Module Requirements/EA4 Specific/ES320A_MotDrvDiagc)' '#ES320A_192' 'true' 'REQ: ES320A_192' '' } %GIDa_41e9d3d1_2cbe_426a_a253_f7bdfc7fddd5  TreatAsAtomicUnit=on
  Copyright1 : Subsystem  Description=|  RequirementInfo={} %GIDa_4a7833ac_b8ea_4821_8ab2_f100b11f2d64  mask(Copyright Information){none=on}
      | Copyright info block.                                               
      |                                                                     
      | Place copyright information at the top of every subsystem in design.
      mask prompts: none "No parameters"
      mask help: Place copyright information at the top of every subsystem in design.
      mask Display:
      | NxtrConf = 'Nexteer Confidential';
      | 
      | sys = bdroot; %handle for the current model ("system")
      | first = get_param(sys,'Created');
      | if(isempty(first))
      |     first = datestr(now,'yyyy');
      | else
      |     first = first(end-3:end);  %year is last four digits
      | end
      | 
      | last = get_param(sys,'LastModifiedDate');
      | if isempty(last)
      |     last = datestr(now,'yyyy');
      | else
      |     last = last(end-3:end);
      | end
      | 
      | if strcmp(first,last)
      |     fprintf('%s\nCopyright  %s Nexteer',NxtrConf,first);
      | else
      |     fprintf('%s\n%s%s-%s Nexteer',NxtrConf,char(169),first,last);
      | end
  If : If  IfExpression=u1
  Merge : Merge
  Relational Operator : RelationalOperator  Operator=<  OutDataTypeStr=boolean
  BitSetB : Outport
  wires:
  BitsetStsB/1(bitsetB) -> Merge/1
  BitsetStsB1/1(bitsetB) -> Merge/2
  Merge/1 -> BitSetB/1
  If/1 -> BitsetStsB/Action
  If/2 -> BitsetStsB1/Action
  Relational Operator/1 -> If/1
  PhaOnTiMeasdB/1 -> Relational Operator/1
  PhaOnTiSumBExp/1 -> Relational Operator/2

== system ES320A_MotDrvDiagc/MotDrvDiagc/MotDrvDiagcPer1/MotDrvDiagcFltChk/MeasdPhaFltChkABC/NtcStInfoPhaB/DetermineBitsetB1 ==
  Action Port : ActionPort  ActionType=else
  Constant5 : Constant  Value=0  OutDataTypeStr=uint8
  Copyright1 : Subsystem  Description=|  RequirementInfo={} %GIDa_6eeacd07_32ef_4d92_80bc_c6c69b1b0a8d  mask(Copyright Information){none=on}
      | Copyright info block.                                               
      |                                                                     
      | Place copyright information at the top of every subsystem in design.
      mask prompts: none "No parameters"
      mask help: Place copyright information at the top of every subsystem in design.
      mask Display:
      | NxtrConf = 'Nexteer Confidential';
      | 
      | sys = bdroot; %handle for the current model ("system")
      | first = get_param(sys,'Created');
      | if(isempty(first))
      |     first = datestr(now,'yyyy');
      | else
      |     first = first(end-3:end);  %year is last four digits
      | end
      | 
      | last = get_param(sys,'LastModifiedDate');
      | if isempty(last)
      |     last = datestr(now,'yyyy');
      | else
      |     last = last(end-3:end);
      | end
      | 
      | if strcmp(first,last)
      |     fprintf('%s\nCopyright  %s Nexteer',NxtrConf,first);
      | else
      |     fprintf('%s\n%s%s-%s Nexteer',NxtrConf,char(169),first,last);
      | end
  BitSetB : Outport
  wires:
  Constant5/1 -> BitSetB/1

== system ES320A_MotDrvDiagc/MotDrvDiagc/MotDrvDiagcPer1/MotDrvDiagcFltChk/MeasdPhaFltChkABC/NtcStInfoPhaC/Copyright1 ==

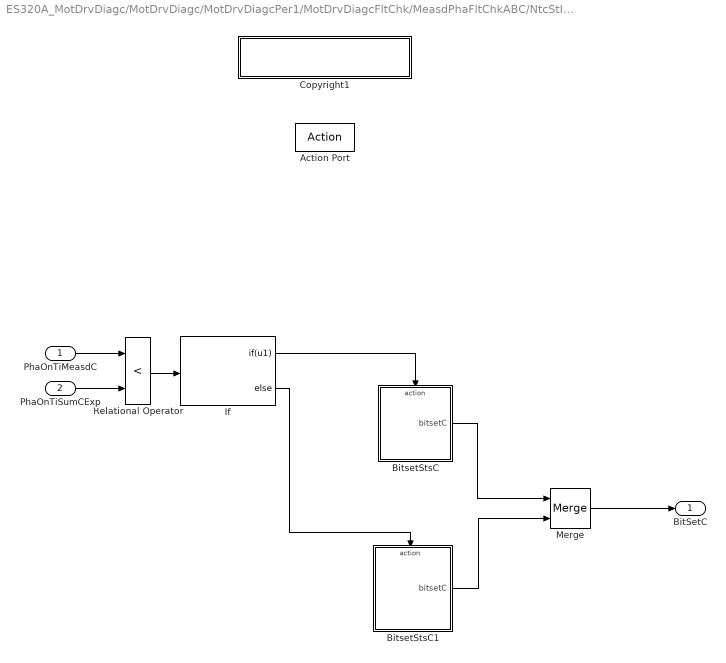
== system ES320A_MotDrvDiagc/MotDrvDiagc/MotDrvDiagcPer1/MotDrvDiagcFltChk/MeasdPhaFltChkABC/NtcStInfoPhaC/DetermineBitsetC ==
  PhaOnTiMeasdC : Inport
  PhaOnTiSumCExp : Inport  Port=2
  Action Port : ActionPort  ActionType=then
  BitsetStsC : Subsystem  RequirementInfo={'linktype_rmi_doors' '0000cf4c (/ESG Group/FDD Module Requirements/EA4 Specific/ES320A_MotDrvDiagc)' '#ES320A_191' 'true' 'REQ: ES320A_191' '' } %GIDa_7028144c_78c0_4c06_af55_d039bdb3ddb3  TreatAsAtomicUnit=on
  BitsetStsC1 : Subsystem  RequirementInfo={'linktype_rmi_doors' '0000cf4c (/ESG Group/FDD Module Requirements/EA4 Specific/ES320A_MotDrvDiagc)' '#ES320A_190' 'true' 'REQ: ES320A_190' '' } %GIDa_a2ccbd9c_dbf4_4e34_b0ab_df59b426f410  TreatAsAtomicUnit=on
  Copyright1 : Subsystem  Description=|  RequirementInfo={} %GIDa_8647a085_3e53_4cb0_92a5_ed3dfaf24295  mask(Copyright Information){none=on}
      | Copyright info block.                                               
      |                                                                     
      | Place copyright information at the top of every subsystem in design.
      mask prompts: none "No parameters"
      mask help: Place copyright information at the top of every subsystem in design.
      mask Display:
      | NxtrConf = 'Nexteer Confidential';
      | 
      | sys = bdroot; %handle for the current model ("system")
      | first = get_param(sys,'Created');
      | if(isempty(first))
      |     first = datestr(now,'yyyy');
      | else
      |     first = first(end-3:end);  %year is last four digits
      | end
      | 
      | last = get_param(sys,'LastModifiedDate');
      | if isempty(last)
      |     last = datestr(now,'yyyy');
      | else
      |     last = last(end-3:end);
      | end
      | 
      | if strcmp(first,last)
      |     fprintf('%s\nCopyright  %s Nexteer',NxtrConf,first);
      | else
      |     fprintf('%s\n%s%s-%s Nexteer',NxtrConf,char(169),first,last);
      | end
  If : If  IfExpression=u1
  Merge : Merge
  Relational Operator : RelationalOperator  Operator=<  OutDataTypeStr=boolean
  BitSetC : Outport
  wires:
  BitsetStsC/1(bitsetC) -> Merge/1
  BitsetStsC1/1(bitsetC) -> Merge/2
  Merge/1 -> BitSetC/1
  If/1 -> BitsetStsC/Action
  If/2 -> BitsetStsC1/Action
  Relational Operator/1 -> If/1
  PhaOnTiMeasdC/1 -> Relational Operator/1
  PhaOnTiSumCExp/1 -> Relational Operator/2
